simulink model "gmStateSpaceHDL_HalfWaveRectifier_HDL"  (R2020b)
settings: Solver=FixedStepDiscrete  StartTime=0.0  StopTime=5*tin  RelTol=1e-3  AbsTol=1e-3
InitFcn:
  | ts = 1e-6; % local solver sample time
  | tin = 100*ts; % input time period
  | load('/home/ts/Dokumente/ultrazohm_testbench/ultrazohm_test/ultrazohm_sw/ip_cores/simscapeHDL_example_v1_0/sschdl/HalfWaveRectifier_HDL/stateSpaceParameters.mat');
undefined symbols (not defined in the file): stateSpaceParameters_1
libraries: simulink x7, hdlssclib x3
CloseFcn:
  | clear ts tin;
settings Model: DataTypeOverride=Off  Creator=The MathWorks, Inc.  LastModifiedBy=ts
settings SolverCC: AutoScaleAbsTol=off
settings DataIOCC: SaveOutput=off  SaveTime=off  ReturnWorkspaceOutputs=off
settings OptimizationCC: BlockReduction=off  ConditionallyExecuteInputs=off  DefaultParameterBehavior=Inlined
settings DebuggingCC: AlgebraicLoopMsg=error  SingleTaskRateTransMsg=error  PregeneratedLibrarySubsystemCodeDiagnostic=none  ArithmeticOperatorsInVariantConditions=warning
settings HardwareCC: ProdBitPerPointer=32  ProdBitPerSizeT=32  ProdBitPerPtrDiffT=32  ProdLargestAtomicFloat=None  ProdIntDivRoundTo=Undefined  ProdEndianess=Unspecified  ProdWordSize=32  ProdHWDeviceType=ASIC/FPGA->ASIC/FPGA  TargetBitPerLong=64  TargetBitPerPointer=64  TargetBitPerSizeT=64  TargetBitPerPtrDiffT=64  TargetLongLongMode=on  TargetIntDivRoundTo=Zero  TargetEndianess=LittleEndian  TargetWordSize=64  TargetHWDeviceType=Custom Processor->MATLAB Host Computer  ProdEqTarget=off
settings SFSimCC: SimUseLocalCustomCode=off  CustomCodeUndefinedFunction=UseInterfaceOnly
settings RTWCC: RTWUseLocalCustomCode=off
settings CodeAppCC: StateflowObjectComments=on
settings SimscapeCC: SimscapeNormalizeSystem=off  SimscapeNominalValues="[{\"value\":\"10\",\"unit\":\"V\"},{\"value\":\"1\",\"unit\":\"A\"},{\"value\":\"10\",\"unit\":\"N*m\"},{\"value\":\"10\",\"unit\":\"bar\"},{\"value\":\"100\",\"unit\":\"kJ/kg\"},{\"value\":\"1\",\"unit\":\"kW\"},{\"value\":\"300\",\"unit\":\"K\"},{\"value\":\"100\",\"unit\":\"cm^3/s\"},{\"value\":\"1\",\"unit\":\"kN\"},{\"value\":\"1\",\"unit\":\"g/cm^3\"},{\"value\":\"1\",\"unit\":\"l\"},{\"value\":\"1\",\"unit\":\"cm^2\"},{\"value\":\"60\",\"unit\":\"Hz\"}]"  SimscapeLogType=all  SimscapeLogDataHistory=10000

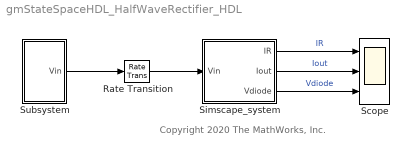
== system gmStateSpaceHDL_HalfWaveRectifier_HDL ==
  note: Copyright 2020 The MathWorks, Inc.
  Rate Transition : RateTransition
  Scope : Scope  NumInputPorts=3
  Simscape_system : Subsystem  TreatAsAtomicUnit=on
  Subsystem : Subsystem
  wires:
  Simscape_system/1(IR) -> Scope/1  "IR"
  Simscape_system/2(Iout) -> Scope/2  "Iout"
  Simscape_system/3(Vdiode) -> Scope/3  "Vdiode"
  Rate Transition/1 -> Simscape_system/1(Vin)
  Subsystem/1(Vin) -> Rate Transition/1

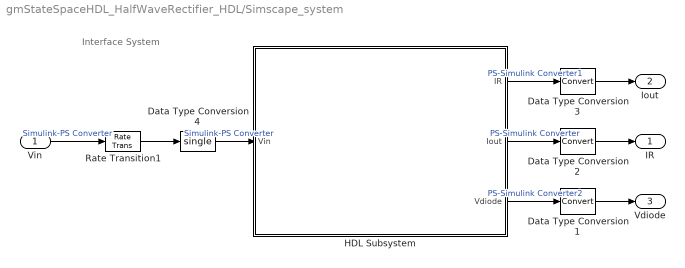
== system gmStateSpaceHDL_HalfWaveRectifier_HDL/Simscape_system ==
  note: Interface System
  Vin : Inport
  Data Type Conversion1 : DataTypeConversion
  Data Type Conversion2 : DataTypeConversion
  Data Type Conversion3 : DataTypeConversion
  Data Type Conversion4 : DataTypeConversion  OutDataTypeStr=single
  HDL Subsystem : Subsystem  TreatAsAtomicUnit=on
  Rate Transition1 : RateTransition  OutPortSampleTime=1e-06
  IR : Outport  VectorParamsAs1DForOutWhenUnconnected=off
  Iout : Outport  Port=2  VectorParamsAs1DForOutWhenUnconnected=off
  Vdiode : Outport  Port=3  VectorParamsAs1DForOutWhenUnconnected=off
  wires:
  Data Type Conversion2/1 -> IR/1
  Data Type Conversion3/1 -> Iout/1
  Rate Transition1/1 -> Data Type Conversion4/1
  Data Type Conversion1/1 -> Vdiode/1
  Data Type Conversion4/1 -> HDL Subsystem/1(Vin)  "Simulink-PS Converter"
  HDL Subsystem/3(Vdiode) -> Data Type Conversion1/1  "PS-Simulink Converter2"
  HDL Subsystem/2(Iout) -> Data Type Conversion2/1  "PS-Simulink Converter"
  HDL Subsystem/1(IR) -> Data Type Conversion3/1  "PS-Simulink Converter1"
  Vin/1 -> Rate Transition1/1  "Simulink-PS Converter"

== system gmStateSpaceHDL_HalfWaveRectifier_HDL/Subsystem ==
  Sine Wave : Sin  Amplitude=10  Frequency=2*pi/(tin)  SampleTime=0
  Vin : Outport  VectorParamsAs1DForOutWhenUnconnected=off
  wires:
  Sine Wave/1 -> Vin/1  "Vin"

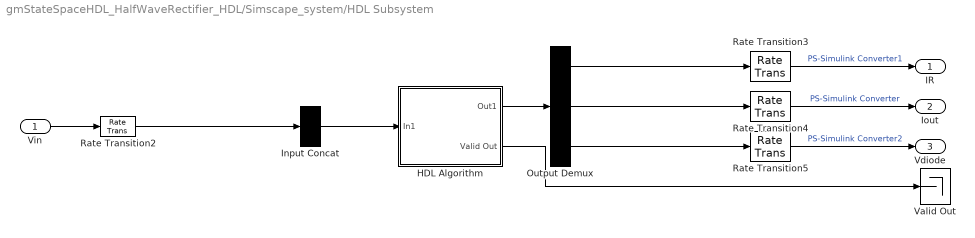
== system gmStateSpaceHDL_HalfWaveRectifier_HDL/Simscape_system/HDL Subsystem ==
  Vin : Inport
  HDL Algorithm : Subsystem
  Input Concat : Concatenate  NumInputs=1
  Output Demux : Demux  Outputs=3
  Rate Transition2 : RateTransition  Integrity=off  OutPortSampleTimeOpt=Multiple of input port sample time  OutPortSampleTimeMultiple=1/3
  Rate Transition3 : RateTransition  OutPortSampleTimeOpt=Multiple of input port sample time  OutPortSampleTimeMultiple=3
  Rate Transition4 : RateTransition  OutPortSampleTimeOpt=Multiple of input port sample time  OutPortSampleTimeMultiple=3
  Rate Transition5 : RateTransition  OutPortSampleTimeOpt=Multiple of input port sample time  OutPortSampleTimeMultiple=3
  Valid Out : Terminator
  IR : Outport
  Iout : Outport  Port=2
  Vdiode : Outport  Port=3
  wires:
  HDL Algorithm/2(Valid Out) -> Valid Out/1
  Output Demux/2 -> Rate Transition4/1
  HDL Algorithm/1(Out1) -> Output Demux/1
  Rate Transition3/1 -> IR/1  "PS-Simulink Converter1"
  Input Concat/1 -> HDL Algorithm/1(In1)
  Rate Transition2/1 -> Input Concat/1
  Rate Transition5/1 -> Vdiode/1  "PS-Simulink Converter2"
  Vin/1 -> Rate Transition2/1
  Output Demux/3 -> Rate Transition5/1
  Rate Transition4/1 -> Iout/1  "PS-Simulink Converter"
  Output Demux/1 -> Rate Transition3/1

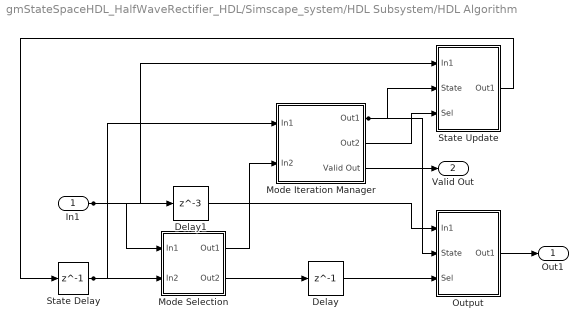
== system gmStateSpaceHDL_HalfWaveRectifier_HDL/Simscape_system/HDL Subsystem/HDL Algorithm ==
  In1 : Inport
  Delay : Delay  DelayLength=1
  Delay1 : Delay  DelayLength=3
  Mode Iteration Manager : Subsystem
  Mode Selection : Subsystem
  Output : Subsystem
  State Delay : Delay  DelayLength=1  InitialCondition=single(stateSpaceParameters_1.X0)
  State Update : Subsystem
  Out1 : Outport  VectorParamsAs1DForOutWhenUnconnected=off
  Valid Out : Outport  Port=2  VectorParamsAs1DForOutWhenUnconnected=off
  wires:
  State Delay/1 -> Mode Selection/2(In2), Mode Iteration Manager/1(In1)
  Mode Iteration Manager/3(Valid Out) -> Valid Out/1
  Delay1/1 -> Output/1(In1)
  In1/1 -> Mode Selection/1(In1), State Update/1(In1), Delay1/1
  Delay/1 -> Output/3(Sel)
  Output/1(Out1) -> Out1/1
  Mode Selection/2(Out2) -> Delay/1
  Mode Iteration Manager/2(Out2) -> State Update/3(Sel)
  Mode Selection/1(Out1) -> Mode Iteration Manager/2(In2)
  Mode Iteration Manager/1(Out1) -> Output/2(State), State Update/2(State)
  State Update/1(Out1) -> State Delay/1

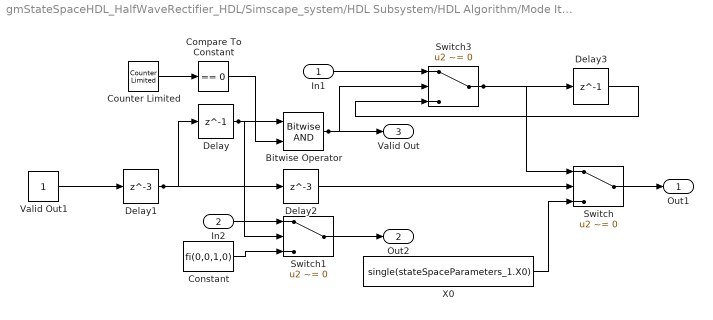
== system gmStateSpaceHDL_HalfWaveRectifier_HDL/Simscape_system/HDL Subsystem/HDL Algorithm/Mode Iteration Manager ==
  In1 : Inport
  In2 : Inport  Port=2
  Bitwise Operator : simulink/Logic and Bit Operations/Bitwise Operator  logicop=AND  UseBitMask=off  NumInputPorts=2  BitMask=bin2dec('11011001')  BitMaskRealWorld=Stored Integer
  Compare To Constant : simulink/Logic and Bit Operations/Compare To Constant  relop===  const=0  OutDataTypeStr=boolean
  Constant : Constant  Value=fi(0,0,1,0)  SampleTime=3.333333333333333e-07
  Counter Limited : simulink/Sources/Counter Limited  uplimit=2  tsamp=-1
  Delay : Delay  DelayLength=1
  Delay1 : Delay  DelayLength=3
  Delay2 : Delay  DelayLength=3
  Delay3 : Delay  DelayLength=1
  Switch : Switch  Criteria=u2 ~= 0
  Switch1 : Switch  Criteria=u2 ~= 0
  Switch3 : Switch  Criteria=u2 ~= 0
  Valid Out1 : Constant  OutDataTypeStr=boolean  SampleTime=3.333333333333333e-07
  X0 : Constant  Value=single(stateSpaceParameters_1.X0)  SampleTime=3.333333333333333e-07
  Out1 : Outport  OutDataTypeStr=single  VectorParamsAs1DForOutWhenUnconnected=off
  Out2 : Outport  Port=2  VectorParamsAs1DForOutWhenUnconnected=off
  Valid Out : Outport  Port=3  VectorParamsAs1DForOutWhenUnconnected=off
  wires:
  Delay1/1 -> Delay2/1, Delay/1
  Bitwise Operator/1 -> Valid Out/1, Switch3/2
  Delay2/1 -> Switch/2
  X0/1 -> Switch/3
  Constant/1 -> Switch1/3
  Switch3/1 -> Delay3/1, Switch/1
  Switch/1 -> Out1/1
  Delay/1 -> Switch1/2, Bitwise Operator/1
  In1/1 -> Switch3/1
  Valid Out1/1 -> Delay1/1
  Delay3/1 -> Switch3/3
  Compare To Constant/1 -> Bitwise Operator/2
  Counter Limited/1 -> Compare To Constant/1
  In2/1 -> Switch1/1
  Switch1/1 -> Out2/1

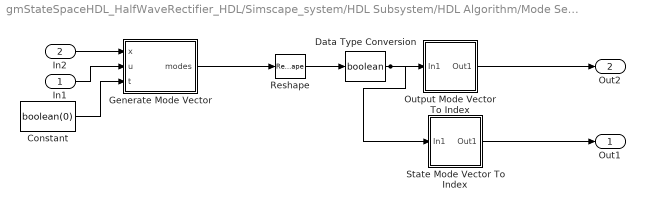
== system gmStateSpaceHDL_HalfWaveRectifier_HDL/Simscape_system/HDL Subsystem/HDL Algorithm/Mode Selection ==
  In1 : Inport
  In2 : Inport  Port=2
  Constant : Constant  Value=boolean(0)  SampleTime=3.333333333333333e-07
  Data Type Conversion : DataTypeConversion  OutDataTypeStr=boolean
  Generate Mode Vector : MATLAB Function  TreatAsAtomicUnit=on
  Output Mode Vector To Index : Subsystem
  Reshape : Reshape
  State Mode Vector To Index : Subsystem
  Out1 : Outport  VectorParamsAs1DForOutWhenUnconnected=off
  Out2 : Outport  Port=2  VectorParamsAs1DForOutWhenUnconnected=off
  wires:
  Data Type Conversion/1 -> State Mode Vector To Index/1(In1), Output Mode Vector To Index/1(In1)
  In1/1 -> Generate Mode Vector/2(u)
  State Mode Vector To Index/1(Out1) -> Out1/1
  Output Mode Vector To Index/1(Out1) -> Out2/1
  Generate Mode Vector/1(modes) -> Reshape/1
  Constant/1 -> Generate Mode Vector/3(t)
  Reshape/1 -> Data Type Conversion/1
  In2/1 -> Generate Mode Vector/1(x)

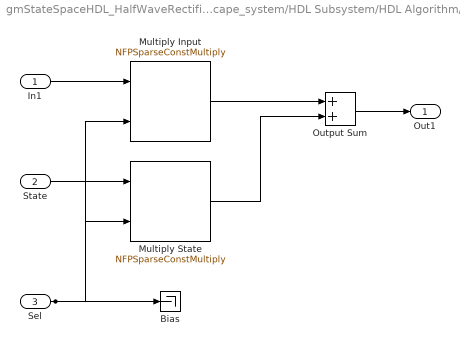
== system gmStateSpaceHDL_HalfWaveRectifier_HDL/Simscape_system/HDL Subsystem/HDL Algorithm/Output ==
  In1 : Inport
  State : Inport  Port=2
  Sel : Inport  Port=3
  Bias : Terminator
  Multiply Input : hdlssclib/NFPSparseConstMultiply  constMatrix=single(stateSpaceParameters_1.Dd)
      settings: SourceProductBaseCode=SL
  Multiply State : hdlssclib/NFPSparseConstMultiply  constMatrix=single(stateSpaceParameters_1.Cd)
      settings: SourceProductBaseCode=SL
  Output Sum : Sum
  Out1 : Outport  VectorParamsAs1DForOutWhenUnconnected=off
  wires:
  State/1 -> Multiply State/1
  In1/1 -> Multiply Input/1
  Sel/1 -> Bias/1, Multiply State/2, Multiply Input/2
  Output Sum/1 -> Out1/1
  Multiply Input/1 -> Output Sum/1
  Multiply State/1 -> Output Sum/2

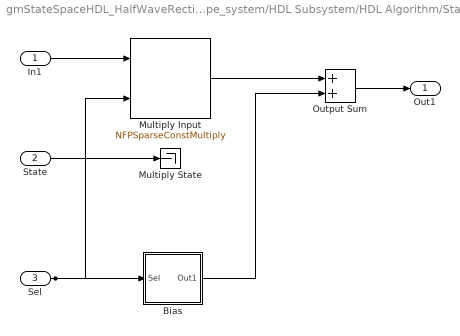
== system gmStateSpaceHDL_HalfWaveRectifier_HDL/Simscape_system/HDL Subsystem/HDL Algorithm/State Update ==
  In1 : Inport
  State : Inport  Port=2
  Sel : Inport  Port=3
  Bias : Subsystem
  Multiply Input : hdlssclib/NFPSparseConstMultiply  constMatrix=single(stateSpaceParameters_1.Bd)
      settings: SourceProductBaseCode=SL
  Multiply State : Terminator
  Output Sum : Sum
  Out1 : Outport  OutDataTypeStr=single  VectorParamsAs1DForOutWhenUnconnected=off
  wires:
  State/1 -> Multiply State/1
  In1/1 -> Multiply Input/1
  Sel/1 -> Bias/1(Sel), Multiply Input/2
  Output Sum/1 -> Out1/1
  Multiply Input/1 -> Output Sum/1
  Bias/1(Out1) -> Output Sum/2

== system gmStateSpaceHDL_HalfWaveRectifier_HDL/Simscape_system/HDL Subsystem/HDL Algorithm/Mode Selection/Output Mode Vector To Index ==
  In1 : Inport
  Index : Constant  Value=fi(0,0,1,0)  SampleTime=3.333333333333333e-07
  Term : Terminator
  Out1 : Outport  VectorParamsAs1DForOutWhenUnconnected=off
  wires:
  In1/1 -> Term/1
  Index/1 -> Out1/1

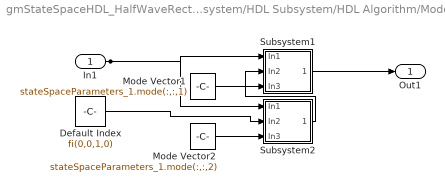
== system gmStateSpaceHDL_HalfWaveRectifier_HDL/Simscape_system/HDL Subsystem/HDL Algorithm/Mode Selection/State Mode Vector To Index ==
  In1 : Inport
  Default Index : Constant  Value=fi(0,0,1,0)  SampleTime=3.333333333333333e-07
  Mode Vector1 : Constant  Value=stateSpaceParameters_1.mode(:,:,1)  OutDataTypeStr=boolean  SampleTime=3.333333333333333e-07
  Mode Vector2 : Constant  Value=stateSpaceParameters_1.mode(:,:,2)  OutDataTypeStr=boolean  SampleTime=3.333333333333333e-07
  Subsystem1 : Subsystem  TreatAsAtomicUnit=on  mask{Index=fi(0,0,1,0)}
  Subsystem2 : Subsystem  TreatAsAtomicUnit=on  mask{Index=fi(1,0,1,0)}
  Out1 : Outport  VectorParamsAs1DForOutWhenUnconnected=off
  wires:
  Mode Vector1/1 -> Subsystem1/3(In3)
  Mode Vector2/1 -> Subsystem2/3(In3)
  In1/1 -> Subsystem1/1(In1), Subsystem2/1(In1)
  Subsystem2/1(Out1) -> Subsystem1/2(In2)
  Subsystem1/1(Out1) -> Out1/1
  Default Index/1 -> Subsystem2/2(In2)

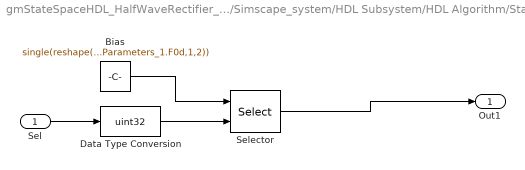
== system gmStateSpaceHDL_HalfWaveRectifier_HDL/Simscape_system/HDL Subsystem/HDL Algorithm/State Update/Bias ==
  Sel : Inport
  Bias : Constant  Value=single(reshape(stateSpaceParameters_1.F0d,1,2))  SampleTime=3.333333333333333e-07
  Data Type Conversion : DataTypeConversion  OutDataTypeStr=uint32
  Selector : Selector  NumberOfDimensions=2  IndexMode=Zero-based  InputPortWidth=3  IndexOptions=Select all,Index vector (port)  Indices=[1 3]  OutputSizes=1
  Out1 : Outport  VectorParamsAs1DForOutWhenUnconnected=off
  wires:
  Bias/1 -> Selector/1
  Sel/1 -> Data Type Conversion/1
  Data Type Conversion/1 -> Selector/2
  Selector/1 -> Out1/1

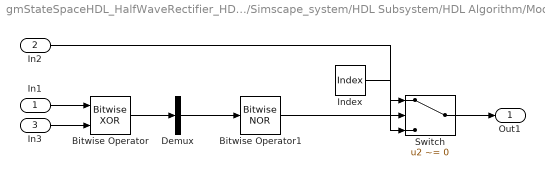
== system gmStateSpaceHDL_HalfWaveRectifier_HDL/Simscape_system/HDL Subsystem/HDL Algorithm/Mode Selection/State Mode Vector To Index/Subsystem1 ==
  In1 : Inport
  In2 : Inport  Port=2
  In3 : Inport  Port=3
  Bitwise Operator : simulink/Logic and Bit Operations/Bitwise Operator  logicop=XOR  UseBitMask=off  NumInputPorts=2  BitMask=bin2dec('11011001')  BitMaskRealWorld=Stored Integer
  Bitwise Operator1 : simulink/Logic and Bit Operations/Bitwise Operator  logicop=NOR  UseBitMask=off  BitMask=bin2dec('11011001')  BitMaskRealWorld=Stored Integer
  Demux : Demux  Outputs=1
  Index : Constant  Value=Index  SampleTime=3.333333333333333e-07
  Switch : Switch  Criteria=u2 ~= 0
  Out1 : Outport  VectorParamsAs1DForOutWhenUnconnected=off
  wires:
  In1/1 -> Bitwise Operator/1
  In3/1 -> Bitwise Operator/2
  Bitwise Operator/1 -> Demux/1
  Demux/1 -> Bitwise Operator1/1
  In2/1 -> Switch/3
  Bitwise Operator1/1 -> Switch/2
  Switch/1 -> Out1/1
  Index/1 -> Switch/1

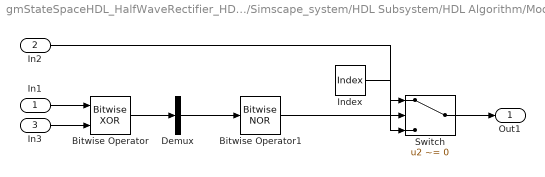
== system gmStateSpaceHDL_HalfWaveRectifier_HDL/Simscape_system/HDL Subsystem/HDL Algorithm/Mode Selection/State Mode Vector To Index/Subsystem2 ==
  In1 : Inport
  In2 : Inport  Port=2
  In3 : Inport  Port=3
  Bitwise Operator : simulink/Logic and Bit Operations/Bitwise Operator  logicop=XOR  UseBitMask=off  NumInputPorts=2  BitMask=bin2dec('11011001')  BitMaskRealWorld=Stored Integer
  Bitwise Operator1 : simulink/Logic and Bit Operations/Bitwise Operator  logicop=NOR  UseBitMask=off  BitMask=bin2dec('11011001')  BitMaskRealWorld=Stored Integer
  Demux : Demux  Outputs=1
  Index : Constant  Value=Index  SampleTime=3.333333333333333e-07
  Switch : Switch  Criteria=u2 ~= 0
  Out1 : Outport  VectorParamsAs1DForOutWhenUnconnected=off
  wires:
  In1/1 -> Bitwise Operator/1
  In3/1 -> Bitwise Operator/2
  Bitwise Operator/1 -> Demux/1
  Demux/1 -> Bitwise Operator1/1
  In2/1 -> Switch/3
  Bitwise Operator1/1 -> Switch/2
  Switch/1 -> Out1/1
  Index/1 -> Switch/1

== matlab function gmStateSpaceHDL_HalfWaveRectifier_HDL/Simscape_system/HDL Subsystem/HDL Algorithm/Mode Selection/Generate Mode Vector ==
  data: x input; u input; modes output; t input
function modes = compute_modes(x,u,t)


  mode1 = (x(1) > (1.0));

  modes = [mode1];

end
